simulink model "TankFuzzy"  (R2014b)
settings: Solver=ode45  SolverMode=SingleTasking  StartTime=0.0  StopTime=600  RelTol=1e-3
values from neighbouring files (symbols this model uses):
  a1 = 0.178    [AG_F_MAM_RULES.m]
  A1 = 15.518    [AG_F_MAM_RULES.m]
  A2 = A1 + 3e-5    (= 15.51803)    [AG_F_MAM_RULES.m]
  a2 = a1+500e-5    (= 0.183)    [AG_F_MAM_RULES.m]
  Fuzzy = Fuzzy_otimo    [AG_F_MAM_RULES.m]
  g = 981    [AG_F_MAM_RULES.m]
  Km = 4.6    [AG_F_MAM_RULES.m]
  L0 = [0;0]    [AG_F_MAM_RULES.m]
libraries: simulink x7, fuzblock x1
settings Model: Creator=Welisson Moura  LastModifiedBy=jeanmarioml
settings DebuggingCC: MaxConsecutiveZCsMsg=none

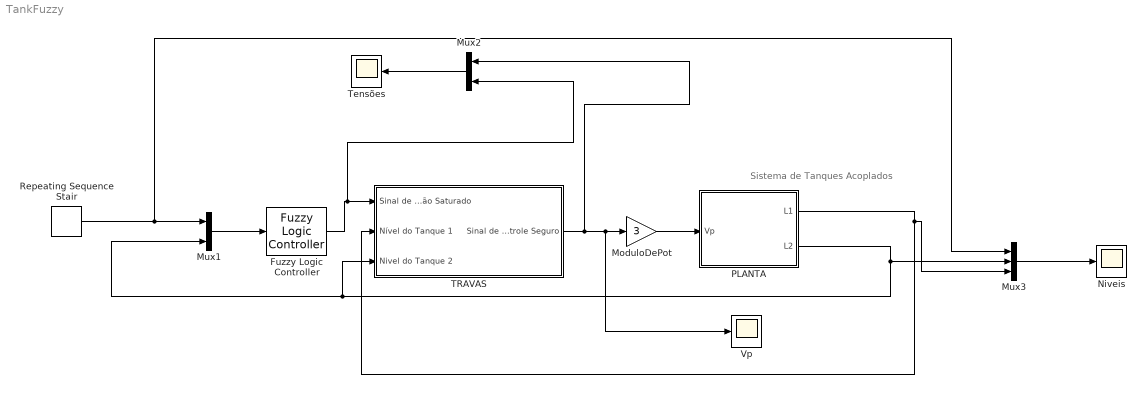
== system TankFuzzy ==
  note: Sistema de Tanques Acoplados
  Fuzzy Logic Controller : fuzblock/Fuzzy Logic  Controller  fis=[Fuzzy]
  ModuloDePot : Gain  Gain=3
  Mux1 : Mux  Inputs=2
  Mux2 : Mux  Inputs=2
  Mux3 : Mux  Inputs=3
  Niveis : Scope
      settings: TimeRange=600  YMin=0  YMax=30  SaveName=Niveis  MaxDataPoints=500000  ScrollMode=on
  PLANTA : Subsystem
  Repeating Sequence Stair : simulink/Sources/Repeating Sequence Stair  OutValues=[15 10 20 5].'  tsamp=150  OutMin=[]  OutMax=[]  OutDataTypeStr=double  OutputDataTypeScalingMode=double  OutDataType=fixdt(0,8)  ConRadixGroup=Best Precision: Vector-wise  OutScaling=2^-12
  TRAVAS : Subsystem
  Tensões : Scope
      settings: SaveName=Vp1  MaxDataPoints=500000
  "Vp " : Scope
      settings: SaveName=Vp  MaxDataPoints=500000
  wires:
  Fuzzy Logic Controller/1 -> Mux2/2, TRAVAS/1(Sinal de Controle Não Saturado)
  Mux1/1 -> Fuzzy Logic Controller/1
  PLANTA/2(L2) -> Mux3/2, TRAVAS/3(Nivel do Tanque 2), Mux1/2
  Repeating Sequence Stair/1 -> Mux3/1, Mux1/1
  Mux3/1 -> Niveis/1
  ModuloDePot/1 -> PLANTA/1(Vp)
  PLANTA/1(L1) -> TRAVAS/2(Nível do Tanque 1), Mux3/3
  TRAVAS/1(Sinal de Controle Seguro) -> Mux2/1, "Vp "/1, ModuloDePot/1
  Mux2/1 -> Tensões/1

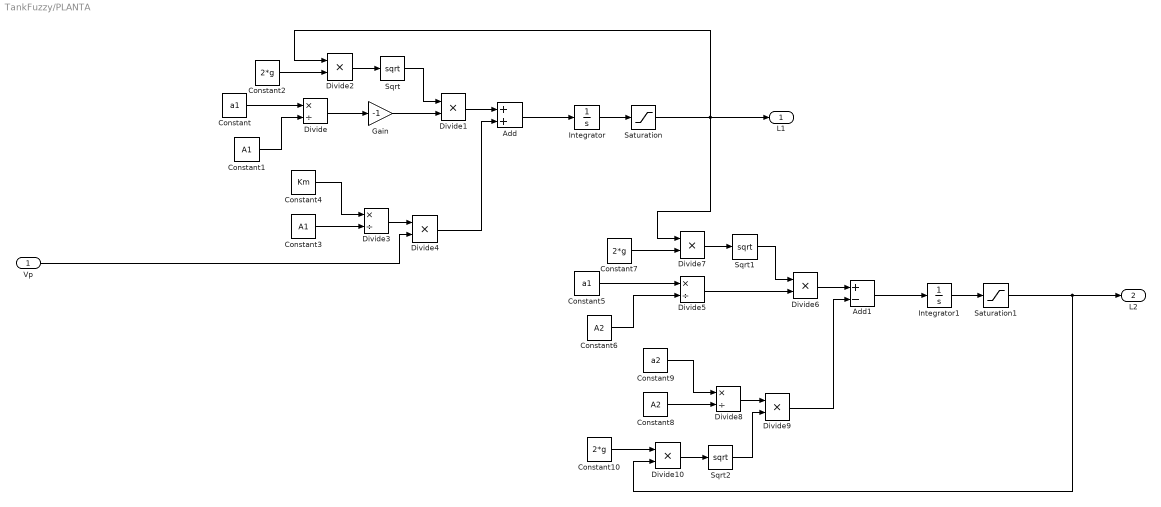
== system TankFuzzy/PLANTA ==
  Vp : Inport
  Add : Sum
  Add1 : Sum  Inputs=+-
  Constant : Constant  Value=a1
  Constant1 : Constant  Value=A1
  Constant10 : Constant  Value=2*g
  Constant2 : Constant  Value=2*g
  Constant3 : Constant  Value=A1
  Constant4 : Constant  Value=Km
  Constant5 : Constant  Value=a1
  Constant6 : Constant  Value=A2
  Constant7 : Constant  Value=2*g
  Constant8 : Constant  Value=A2
  Constant9 : Constant  Value=a2
  Divide{,3,5,8} (4 alike) : Product  Inputs=*/
  Divide{1..2,4,6..7,9..10} (7 alike) : Product  Inputs=**
  Gain : Gain  Gain=-1
  Integrator : Integrator  InitialCondition=L0(1)
  Integrator1 : Integrator  InitialCondition=L0(2)
  Saturation : Saturate  UpperLimit=30  LowerLimit=0  ZeroCross=off
  Saturation1 : Saturate  UpperLimit=30  LowerLimit=0  ZeroCross=off
  Sqrt : Sqrt  SaturateOnIntegerOverflow=on
  Sqrt1 : Sqrt  SaturateOnIntegerOverflow=on
  Sqrt2 : Sqrt  SaturateOnIntegerOverflow=on
  L1 : Outport
  L2 : Outport  Port=2
  wires:
  Constant/1 -> Divide/1
  Constant1/1 -> Divide/2
  Divide/1 -> Gain/1
  Gain/1 -> Divide1/2
  Sqrt/1 -> Divide1/1
  Divide2/1 -> Sqrt/1
  Constant2/1 -> Divide2/2
  Divide1/1 -> Add/1
  Constant3/1 -> Divide3/2
  Constant4/1 -> Divide3/1
  Divide3/1 -> Divide4/1
  Vp/1 -> Divide4/2
  Divide4/1 -> Add/2
  Add/1 -> Integrator/1
  Integrator/1 -> Saturation/1
  Saturation/1 -> Divide2/1, Divide7/1, L1/1
  Constant5/1 -> Divide5/1
  Constant6/1 -> Divide5/2
  Divide5/1 -> Divide6/2
  Sqrt1/1 -> Divide6/1
  Divide7/1 -> Sqrt1/1
  Constant7/1 -> Divide7/2
  Divide6/1 -> Add1/1
  Constant8/1 -> Divide8/2
  Constant9/1 -> Divide8/1
  Divide8/1 -> Divide9/1
  Divide9/1 -> Add1/2
  Add1/1 -> Integrator1/1
  Integrator1/1 -> Saturation1/1
  Saturation1/1 -> Divide10/2, L2/1
  Constant10/1 -> Divide10/1
  Divide10/1 -> Sqrt2/1
  Sqrt2/1 -> Divide9/2

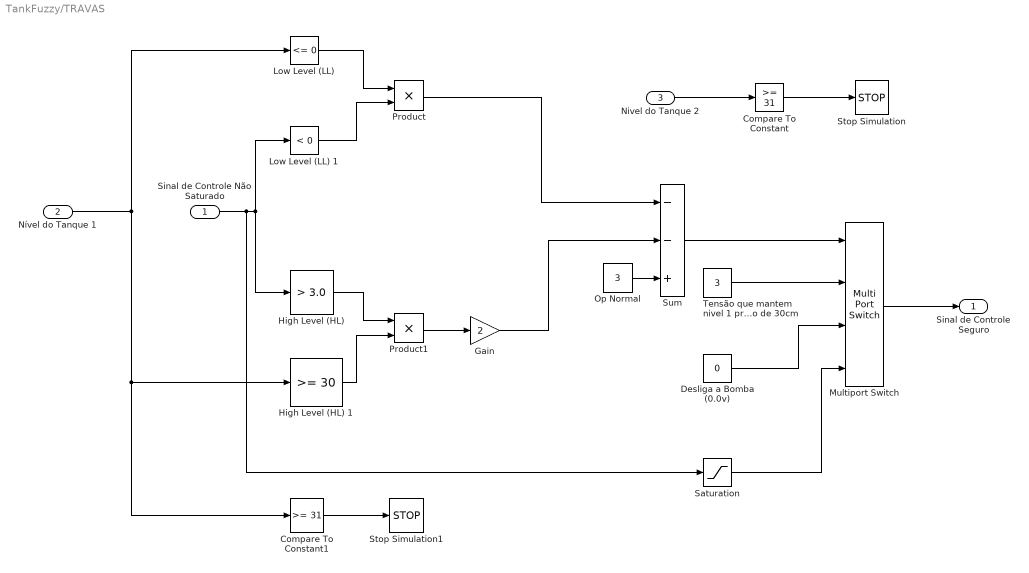
== system TankFuzzy/TRAVAS ==
  Sinal de Controle Não Saturado : Inport
  Nível do Tanque 1 : Inport  Port=2
  Nivel do Tanque 2 : Inport  Port=3
  " High Level (HL) 1" : simulink/Logic and Bit Operations/Compare To Constant  relop=>=  const=30  OutDataTypeStr=boolean  ZeroCross=off
  Compare To Constant : simulink/Logic and Bit Operations/Compare To Constant  relop=>=  const=31  OutDataTypeStr=boolean
  Compare To Constant1 : simulink/Logic and Bit Operations/Compare To Constant  relop=>=  const=31  OutDataTypeStr=boolean
  Desliga a Bomba (0.0v) : Constant  Value=0
  Gain : Gain  Gain=2
  High Level (HL) : simulink/Logic and Bit Operations/Compare To Constant  relop=>  const=3.0  OutDataTypeStr=boolean  ZeroCross=off
  "Low Level (LL) " : simulink/Logic and Bit Operations/Compare To Constant  relop=<=  const=0  OutDataTypeStr=boolean
  "Low Level (LL) 1 " : simulink/Logic and Bit Operations/Compare To Constant  relop=<  const=0  OutDataTypeStr=boolean
  Multiport Switch : MultiPortSwitch
  Op Normal : Constant  Value=3
  Product : Product
  Product1 : Product
  Saturation : Saturate  UpperLimit=4  LowerLimit=-4
  Stop Simulation : Stop
  Stop Simulation1 : Stop
  Sum : Sum  Inputs=--+
  Tensão que mantem nivel 1 proximo de 30cm : Constant  Value=3
  Sinal de Controle Seguro : Outport
  wires:
  Compare To Constant/1 -> Stop Simulation/1
  Nivel do Tanque 2/1 -> Compare To Constant/1
  "Low Level (LL) "/1 -> Product/1
  "Low Level (LL) 1 "/1 -> Product/2
  High Level (HL)/1 -> Product1/1
  " High Level (HL) 1"/1 -> Product1/2
  Product1/1 -> Gain/1
  Compare To Constant1/1 -> Stop Simulation1/1
  Nível do Tanque 1/1 -> "Low Level (LL) "/1, " High Level (HL) 1"/1, Compare To Constant1/1
  Sinal de Controle Não Saturado/1 -> Saturation/1, "Low Level (LL) 1 "/1, High Level (HL)/1
  Op Normal/1 -> Sum/3
  Gain/1 -> Sum/2
  Product/1 -> Sum/1
  Sum/1 -> Multiport Switch/1
  Tensão que mantem nivel 1 proximo de 30cm/1 -> Multiport Switch/2
  Desliga a Bomba (0.0v)/1 -> Multiport Switch/3
  Saturation/1 -> Multiport Switch/4
  Multiport Switch/1 -> Sinal de Controle Seguro/1
